simulink model "cruise"  (Simulink 4.00)
settings: Solver=ode5  StartTime=0.0  StopTime=1500  FixedStep=1.5  RelTol=1e-3
settings Model: Creator=jingcao  LastModifiedBy=jingcao  LimitDataPoints=off  ExtModeTrigMode=oneshot  ExtModeArmWhenConnect=off  ExtModeAutoUpdateStatusClock=off  BlockReductionOpt=off

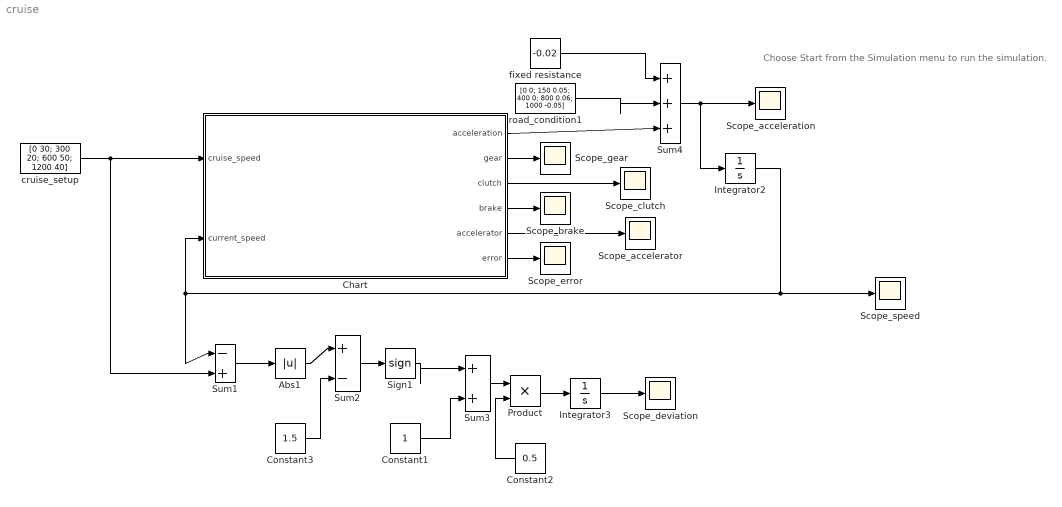
== system cruise ==
  note: Choose Start from
      | the Simulation menu
      | to run the simulation.
  Abs1 : Abs  SaturateOnIntegerOverflow=on
  Chart : Stateflow chart
      settings: RTWFcnNameOpts=Auto  RTWFileNameOpts=Auto
  Constant1 : Constant  Value=1
  Constant2 : Constant  Orientation=left  Value=0.5
  Constant3 : Constant  Value=1.5
  Integrator2 : Integrator  ExternalReset=none  InitialConditionSource=internal  InitialCondition=0  LimitOutput=off  UpperSaturationLimit=inf  LowerSaturationLimit=-inf  ShowSaturationPort=off  ShowStatePort=off  AbsoluteTolerance=auto
  Integrator3 : Integrator  ExternalReset=none  InitialConditionSource=internal  InitialCondition=0  LimitOutput=off  UpperSaturationLimit=inf  LowerSaturationLimit=-inf  ShowSaturationPort=off  ShowStatePort=off  AbsoluteTolerance=auto
  Product : Product  Inputs=2  Multiplication=Element-wise(.*)  SaturateOnIntegerOverflow=on
  Scope_acceleration : Scope
      settings: TimeRange=auto  YMin=0  YMax=80  SaveToWorkspace=off  LimitDataPoints=on  MaxDataPoints=5000
  Scope_accelerator : Scope
      settings: TimeRange=auto  YMin=-6  YMax=3  SaveToWorkspace=off  SaveName=ScopeData4  LimitDataPoints=on  MaxDataPoints=5000
  Scope_brake : Scope
      settings: TimeRange=auto  YMin=-6  YMax=3  SaveToWorkspace=off  SaveName=ScopeData6  LimitDataPoints=on  MaxDataPoints=5000
  Scope_clutch : Scope
      settings: TimeRange=auto  YMin=-6  YMax=3  SaveToWorkspace=off  SaveName=ScopeData2  LimitDataPoints=on  MaxDataPoints=5000
  Scope_deviation : Scope
      settings: TimeRange=auto  YMin=-5  YMax=5  SaveToWorkspace=off  SaveName=ScopeData7  LimitDataPoints=on  MaxDataPoints=5000
  Scope_error : Scope
      settings: TimeRange=auto  YMin=-5  YMax=5  SaveToWorkspace=off  SaveName=ScopeData3  LimitDataPoints=on  MaxDataPoints=5000
  Scope_gear : Scope
      settings: TimeRange=auto  YMin=-6  YMax=3  SaveToWorkspace=off  SaveName=ScopeData5  LimitDataPoints=on  MaxDataPoints=5000
  Scope_speed : Scope
      settings: TimeRange=auto  YMin=0  YMax=80  SaveToWorkspace=off  SaveName=ScopeData  LimitDataPoints=on  MaxDataPoints=5000
  Sign1 : Signum
  Sum1 : Sum  Inputs=|-+  SaturateOnIntegerOverflow=on
  Sum2 : Sum  Inputs=|+-  SaturateOnIntegerOverflow=on
  Sum3 : Sum  Inputs=|++  SaturateOnIntegerOverflow=on
  Sum4 : Sum  Inputs=|+++  SaturateOnIntegerOverflow=on
  cruise_setup : FromWorkspace  VariableName=[0 30; 300 20; 600 50; 1200 40]  SampleTime=0  Interpolate=off  OutputAfterFinalValue=HoldingFinalValue
  fixed resistance : Constant  Value=-0.02
  road_condition1 : FromWorkspace  VariableName=[0 0; 150 0.05; 400 0; 800 0.06; 1000 -0.05]  SampleTime=0  Interpolate=off  OutputAfterFinalValue=HoldingFinalValue
  wires:
  Chart/1(acceleration) -> Sum4/3
  Integrator2/1 -> Sum1/1, Chart/2(current_speed), Scope_speed/1
  Chart/5(accelerator) -> Scope_accelerator/1
  Chart/4(brake) -> Scope_brake/1
  Abs1/1 -> Sum2/1
  Sum2/1 -> Sign1/1
  Sign1/1 -> Sum3/1
  Integrator3/1 -> Scope_deviation/1
  Sum3/1 -> Product/1
  Constant2/1 -> Product/2
  Product/1 -> Integrator3/1
  Constant3/1 -> Sum2/2
  Constant1/1 -> Sum3/2
  fixed resistance/1 -> Sum4/1
  cruise_setup/1 -> Chart/1(cruise_speed), Sum1/2
  Chart/6(error) -> Scope_error/1
  Chart/3(clutch) -> Scope_clutch/1
  Chart/2(gear) -> Scope_gear/1
  road_condition1/1 -> Sum4/2
  Sum4/1 -> Scope_acceleration/1, Integrator2/1
  Sum1/1 -> Abs1/1

== stateflow chart Chart ==
  state Clutch [parallel]
    state released
      en:
      clutch=0;
    state pressed
      en:
      clutch=1;
    released -> pressed : press_clutch
    pressed -> released : release_clutch
    (default) -> released : {clutch=0;}
  state Accelerator [parallel]
    state idle
      en:
    state delay
      en:
      tmp=t+ACCE_DELAY*ml.abs(toAcceLevel-accelerator);
    state adjust
      en:
      accelerator=toAcceLevel;
      tmp=t;
    Accelerator.idle -> Accelerator.delay : adjust_accelerator
    (default) -> Accelerator.idle : /accelerator=0;
    Accelerator.delay -> Accelerator.adjust : [t>tmp]
    Accelerator.adjust -> Accelerator.idle : [t>tmp]
  state Safety_checking2 [parallel]
    state safe
      en:
    state error
      en:error[2]=1;
    Safety_checking2.safe -> (junction 34) : [gear==1&&clutch==0]
    (junction 36) -> Safety_checking2.safe
    Safety_checking2.safe -> (junction 36) : [gear==3&&clutch==0]
    (junction 36) -> Safety_checking2.error : [current_speed<GEAR3MIN]
    Safety_checking2.safe -> (junction 35) : [gear==2&&clutch==0]
    (junction 34) -> Safety_checking2.error : [current_speed<GEAR1MIN]
    (junction 35) -> Safety_checking2.error : [current_speed<GEAR2MIN]
    (default) -> Safety_checking2.safe : {error[2]=0;}
    (junction 34) -> Safety_checking2.safe
    (junction 35) -> Safety_checking2.safe
  state Calculation [parallel]
    state start
      en:tmp=t;
    state calculating
      en:
      tmp = t;
    (default) -> start : {acceleration=0;}
    start -> calculating : [t>tmp]
        | {acceleration=ml.calculate_acceleration(clutch,current_speed, accelerator, gear,brake);}
    calculating -> start : [t>tmp]
  state Gear_state [parallel]
    state third
      en:gear=3;
    state first
      en:gear=1;
    state second
      en:gear=2;
    (default) -> first
    first -> second : shift_up
    second -> first : shift_down
    second -> third : shift_up
    third -> second : shift_down
  state Brake [parallel]
    state delay
      en:
      tmp=t+BRAKE_DELAY*ml.abs(toBrakeLevel-brake);
    state idle
      en:
    state adjust
      en:
      brake=toBrakeLevel;
      tmp=t;
    Brake.idle -> Brake.delay : adjust_brake
    Brake.delay -> Brake.adjust : [t>tmp]
    Brake.adjust -> Brake.idle : [t>tmp]
    (default) -> Brake.idle : /brake=0;
  state Safety_checking3 [parallel]
    state safe
      en:
    state error
      en:error[3]=1;
    Safety_checking3.safe -> Safety_checking3.error : [brake!=0&&accelerator!=0]
    (default) -> Safety_checking3.safe : {error[3]=0;}
  note: 1. To let the cruise controller control the degree of the accelerator, you should first set up the variable
      | toAcceLevel (between 0 to 5) and then fire event adjust_accelerator. There will be certain delay between
      |  you fire the event and the accelerator adapts to the degree that you specified.
      | 2. To let the cruise controller control the brake, you should first set up the variable toBrakeLevel (between
      | 0 and 5) and then fire event adjust_brake. There will be certain delay between you fire the event and the
      | brake adapts to the degree that you specified.
      | 3. The way to control the clutch and select the gear is obvious from the stateflow.
      | 4. You are only allowed to modify  the model of cruise_controller. All the varialbe  that you add should be
      | local to cruise_controller.
  state Safety_checking1 [parallel]
    state safe
    state error
      en:error[1]=1;
    (junction 33) -> Safety_checking1.safe : [clutch==1]
    (junction 33) -> Safety_checking1.error : [clutch==0]
    (default) -> Safety_checking1.safe : {error[1]=0;}
    Safety_checking1.safe -> (junction 32) : shift_up
    (junction 32) -> Safety_checking1.safe : [clutch==1]
    (junction 32) -> Safety_checking1.error : [clutch==0]
    Safety_checking1.safe -> (junction 33) : shift_down
  state Cruise_controller [parallel]
  data: ACCE_DELAY constant =1; tmp local; tmp local double; coef local double; data1 local double; BRAKE_DELAY constant =1; tmp local; cruise_speed input double; current_speed input double; acceleration output double [-100..100]; gear output double =1; clutch output double; brake output double; GEAR1MAX constant double =30; GEAR2MAX constant double =50; GEAR3MAX constant double =70; GEAR1MIN constant double =-10; GEAR2MIN constant double =10; GEAR3MIN constant double =30; accelerator output double; error output double size=3; toAcceLevel local [0..5]; toBrakeLevel local [0..5]
  events: press_clutch local EITHER_EDGE_EVENT; release_clutch local EITHER_EDGE_EVENT; shift_down local EITHER_EDGE_EVENT; shift_up local EITHER_EDGE_EVENT; adjust_accelerator local EITHER_EDGE_EVENT; adjust_brake local EITHER_EDGE_EVENT
